simulink model "teste3"  (R2014a)
settings: Solver=ode45  StartTime=0.0  StopTime=100  RelTol=1e-3
settings Model: Creator=andre  LastModifiedBy=andre
settings DataIOCC: Refine=250

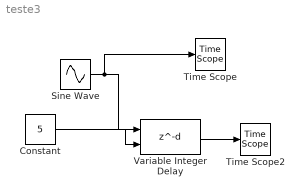
== system teste3 ==
  Constant : Constant  Value=5
  Sine Wave : Sin  Frequency=0.2  Samples=100  SampleTime=0
  Time Scope : TimeScope  DefaultConfigurationName=spbscopes.TimeScopeBlockCfg
  Time Scope2 : TimeScope  DefaultConfigurationName=spbscopes.TimeScopeBlockCfg
  Variable Integer Delay : Delay  DelayLengthSource=Input port
      settings: InputPortMap=u0,p1
  wires:
  Sine Wave/1 -> Variable Integer Delay/1, Time Scope/1
  Variable Integer Delay/1 -> Time Scope2/1
  Constant/1 -> Variable Integer Delay/2
